simulink library "crf"  (Simulink 8.1)
settings: Solver=ode1  StartTime=0.0  StopTime=Inf  FixedStep=0.001  RelTol=1e-3
PostLoadFcn:
  | , if any(exist('dsrtsu_mdlpostloadfcn', 'file') == [2, 3, 6]), try dsrtsu_mdlpostloadfcn('Execute', bdroot); catch fprintf('Error in PostLoadFcn (dsrtsu_mdlpostloadfcn) for model "%s":\n %s\n', bdroot, lasterr); end, end,
undefined symbols (not defined in the file or in its folder): ENUM_PARKBRAKEBINDSTA_RELEASE, KJUD_ACCClearanceToStartMargin_m
settings Model: DSRTSU_INTERNAL_RTI_VER=450  DSRTSU_INTERNAL_RTI_TYPE=rti1401  RTICANMMDATA=struct('GeneralSetupData',struct('modelroot','D:\ELN150201_TAIWAN\trunk\AdasDragon\software\sw_development\arch\app\jud','generalsettings',struct('filesettings',struct('destfolder',struct('Name','RTICANMM_FILES','Check',1),'buildfolder',struct('Name','.','Check',1),'AbsDestfolder',struct('Name','D:\ELN150201_TAIWAN\trunk\AdasDragon\software\sw_development\arch\app\jud\RTICANMM_FILES'),'AbsBuildfolder',struct('Name','D:\ELN150201_TAIWAN\trunk\AdasDragon\software\sw_development\arch\app\jud'))),'options',struct('addpaths',1,'rmpaths',1,'addtrcexclusion',logical(1),'cannavigator',struct('checkmonitoring',0),'show_usrtrc',0,'use_usrtrc',0),'advanced',struct('options',[1 1 1 1 1 1 1 1 1 1 1 1 1 1 1 1 1 1 1 1 1 1 1 1 1 1 1 1 1 1 1 1 1 1 1 1 1 1 1 1 1 1 1 1 1 1 1 1 1 1 1 1 1 1 1 1 1 1 1 1 1 1 1 1 1 1 1 1 1 1 1 1 1 1 1 1 1 1 1 1 1 1 1 1 1 1 1 1 1 1 1 1 1 1 1 1 1 1 1 1]),'MPSetup',{{}},'modelname','crf','block','crf'))  DSRTSU_INTERNAL_RTIFPGA=40  Creator=AT015411  LastModifiedBy=AT015555

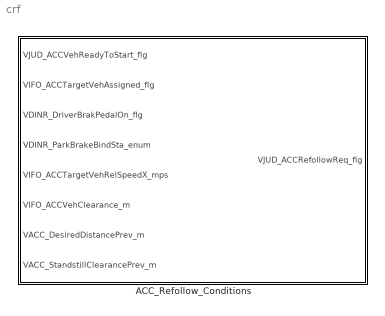
== system crf ==
  ACC_Refollow_Conditions : Subsystem

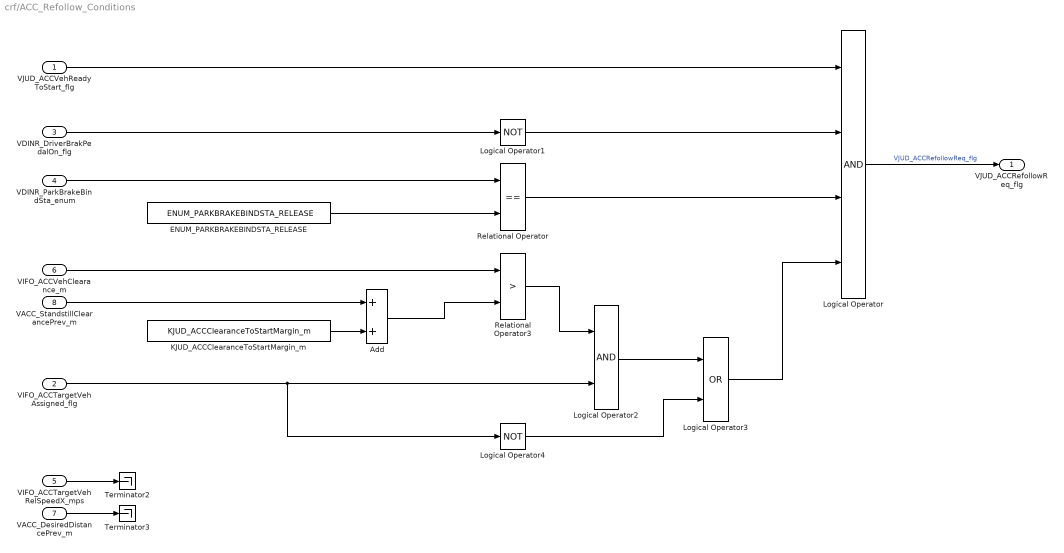
== system crf/ACC_Refollow_Conditions ==
  VJUD_ACCVehReadyToStart_flg : Inport
  VIFO_ACCTargetVehAssigned_flg : Inport  Port=2
  VDINR_DriverBrakPedalOn_flg : Inport  Port=3
  VDINR_ParkBrakeBindSta_enum : Inport  Port=4
  VIFO_ACCTargetVehRelSpeedX_mps : Inport  Port=5
  VIFO_ACCVehClearance_m : Inport  Port=6
  VACC_DesiredDistancePrev_m : Inport  Port=7
  VACC_StandstillClearancePrev_m : Inport  Port=8
  Add : Sum
  ENUM_PARKBRAKEBINDSTA_RELEASE : Constant  Value=ENUM_PARKBRAKEBINDSTA_RELEASE
  KJUD_ACCClearanceToStartMargin_m : Constant  Value=KJUD_ACCClearanceToStartMargin_m
  Logical Operator : Logic  Inputs=4  AllPortsSameDT=off  OutDataTypeStr=boolean
  Logical Operator1 : Logic  Operator=NOT  AllPortsSameDT=off  OutDataTypeStr=boolean
  Logical Operator2 : Logic  AllPortsSameDT=off  OutDataTypeStr=boolean
  Logical Operator3 : Logic  Operator=OR  AllPortsSameDT=off  OutDataTypeStr=boolean
  Logical Operator4 : Logic  Operator=NOT  AllPortsSameDT=off  OutDataTypeStr=boolean
  Relational Operator : RelationalOperator  Operator===  OutDataTypeStr=boolean
  Relational Operator3 : RelationalOperator  Operator=>  OutDataTypeStr=boolean
  Terminator2 : Terminator
  Terminator3 : Terminator
  VJUD_ACCRefollowReq_flg : Outport
  wires:
  Logical Operator/1 -> VJUD_ACCRefollowReq_flg/1  "VJUD_ACCRefollowReq_flg"
  VJUD_ACCVehReadyToStart_flg/1 -> Logical Operator/1
  Logical Operator1/1 -> Logical Operator/2
  VDINR_DriverBrakPedalOn_flg/1 -> Logical Operator1/1
  VDINR_ParkBrakeBindSta_enum/1 -> Relational Operator/1
  Relational Operator/1 -> Logical Operator/3
  ENUM_PARKBRAKEBINDSTA_RELEASE/1 -> Relational Operator/2
  VIFO_ACCTargetVehRelSpeedX_mps/1 -> Terminator2/1
  VIFO_ACCTargetVehAssigned_flg/1 -> Logical Operator4/1, Logical Operator2/2
  Logical Operator2/1 -> Logical Operator3/1
  Logical Operator4/1 -> Logical Operator3/2
  Logical Operator3/1 -> Logical Operator/4
  VIFO_ACCVehClearance_m/1 -> Relational Operator3/1
  VACC_DesiredDistancePrev_m/1 -> Terminator3/1
  KJUD_ACCClearanceToStartMargin_m/1 -> Add/2
  VACC_StandstillClearancePrev_m/1 -> Add/1
  Add/1 -> Relational Operator3/2
  Relational Operator3/1 -> Logical Operator2/1
